simulink model "Controle_fforward"  (R2013a)
settings: Solver=ode45  StartTime=0.0  StopTime=2.0  RelTol=1e-3
undefined symbols (not defined in the file): kukaKR6
libraries: roblocks x4
settings Model: Creator=corkep  LastModifiedBy=Romeu
settings DataIOCC: SignalLoggingSaveFormat=ModelDataLogs
settings OptimizationCC: ExpressionDepthLimit=2147483647
settings DebuggingCC: FcnCallInpInsideContextMsg=UseLocalSettings
settings GRTTargetCC: CombineOutputUpdateFcns=off  GRTInterface=on

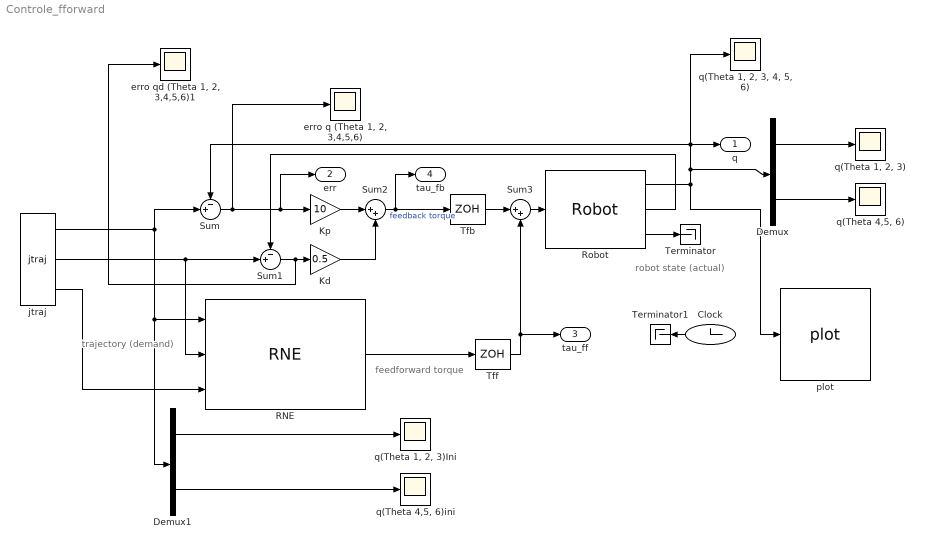
== system Controle_fforward ==
  note: trajectory
      | (demand)
  note: robot state
      | (actual)
  note: feedforward torque
  Clock : Clock
  Demux : Demux  Outputs=2
  Demux1 : Demux  Outputs=2
  Kd : Gain  Gain=0.5  SaturateOnIntegerOverflow=on  OutDataTypeStr=Inherit: Same as input  ParamDataTypeStr=Inherit: Same as input
  Kp : Gain  Gain=10  SaturateOnIntegerOverflow=on  OutDataTypeStr=Inherit: Same as input  ParamDataTypeStr=Inherit: Same as input
  RNE : roblocks/Dynamics/RNE  robot=kukaKR6.nofriction()  grav=[0 0 9.81]
  Robot : roblocks/Dynamics/Robot  robot=kukaKR6  q0=[0 0 0 0 0 0]
  Sum : Sum  Inputs=-+|  SaturateOnIntegerOverflow=on  InputSameDT=on  OutDataTypeStr=Inherit: Same as first input
  Sum1 : Sum  Inputs=-+|  SaturateOnIntegerOverflow=on  InputSameDT=on  OutDataTypeStr=Inherit: Same as first input
  Sum2 : Sum  Inputs=|++  SaturateOnIntegerOverflow=on  InputSameDT=on  OutDataTypeStr=Inherit: Same as first input
  Sum3 : Sum  Inputs=|++  SaturateOnIntegerOverflow=on  InputSameDT=on  OutDataTypeStr=Inherit: Same as first input
  Terminator : Terminator
  Terminator1 : Terminator
  Tfb : ZeroOrderHold  SampleTime=0.01
  Tff : ZeroOrderHold  SampleTime=0.01
  "erro q (Theta 1, 2, 3,4,5,6)" : Scope
      settings: YMin=-0.02  YMax=0.045  SaveName=ScopeData4
  "erro qd (Theta 1, 2, 3,4,5,6)1" : Scope
      settings: TimeRange=2  YMin=-0.0225  YMax=0.025  SaveName=ScopeData5
  jtraj : roblocks/Trajectory/jtraj  q0=[0 0 0 0 0 0]  qf=[pi/2 pi/0.75 -pi/2 0 -pi/4 0]  tmax=2  ts=0.02
  plot : roblocks/Robot Graphics/plot  robot=kukaKR6  fps=25  holdplot=on
  "q(Theta 1, 2, 3)" : Scope
      settings: YMin=-1.1  YMax=1.1  SaveName=ScopeData2
  "q(Theta 1, 2, 3)Ini" : Scope
      settings: YMin=-1  YMax=1
  "q(Theta 1, 2, 3, 4, 5, 6)" : Scope
      settings: YMin=-1.1  YMax=1.1  SaveName=ScopeData6
  "q(Theta 4,5, 6)" : Scope
      settings: YMin=-0.00125  YMax=0.0015
  "q(Theta 4,5, 6)ini" : Scope
      settings: YMin=-0.00025  YMax=0.0004  SaveName=ScopeData3
  q : Outport
  err : Outport  Port=2
  tau_ff : Outport  Port=3
  tau_fb : Outport  Port=4
  wires:
  Kd/1 -> Sum2/2
  Sum/1 -> "erro q (Theta 1, 2, 3,4,5,6)"/1, Kp/1, err/1
  Kp/1 -> Sum2/1
  Sum1/1 -> "erro qd (Theta 1, 2, 3,4,5,6)1"/1, Kd/1
  Sum2/1 -> Tfb/1, tau_fb/1  "feedback torque"
  Sum3/1 -> Robot/1
  Robot/1 -> "q(Theta 1, 2, 3, 4, 5, 6)"/1, q/1, Sum/1, Demux/1, plot/1
  Robot/2 -> Sum1/1
  jtraj/2 -> Sum1/2, RNE/2
  jtraj/3 -> RNE/3
  Robot/3 -> Terminator/1
  Tff/1 -> Sum3/2, tau_ff/1
  Tfb/1 -> Sum3/1
  RNE/1 -> Tff/1
  Clock/1 -> Terminator1/1
  Demux/1 -> "q(Theta 1, 2, 3)"/1
  Demux/2 -> "q(Theta 4,5, 6)"/1
  jtraj/1 -> Demux1/1, RNE/1, Sum/2
  Demux1/1 -> "q(Theta 1, 2, 3)Ini"/1
  Demux1/2 -> "q(Theta 4,5, 6)ini"/1
